simulink model "speedgoat_IO316_100k_21_CI_02826_v2"  (R2023a)
settings: Solver=FixedStepDiscrete  StartTime=0.0  StopTime=inf  RelTol=1e-3
PreLoadFcn:
  | if ~exist('Ts', 'var')
  | Ts = 0.001;
  | end
  | if ~exist('FPGA_Frequency', 'var')
  | FPGA_Frequency = 75000000;
  | end
  | if ~exist('Tpwm', 'var')
  | Tpwm = 0.005;
  | end
undefined symbols (not defined in the file or in its folder): IO316, IO3xx
libraries: simulink x3, speedgoatlib_fpga_pwm x2, speedgoatlib_fpga_dio x2, speedgoatlib_fpga_spi x2, hdlsllib x2, speedgoatlib_fpga_inta x1, speedgoatlib_interrupt x1, speedgoatlib_fpga_quadrature x1, speedgoatlib_fpga x1
settings Model: Creator=jeffrey.gruenig  LastModifiedBy=jeffrey.gruenig
settings SolverCC: ConcurrentTasks=on  PositivePriorityOrder=on
settings DataIOCC: SaveFormat=StructureWithTime
settings OptimizationCC: BlockReduction=off  OptimizeBlockIOStorage=off  BufferReuse=off
settings DebuggingCC: UnderspecifiedInitializationDetection=Classic  MergeDetectMultiDrivingBlocksExec=none  TasksWithSamePriorityMsg=none
settings HardwareCC: ProdBitPerLong=64  ProdLongLongMode=on  ProdHWDeviceType=Intel->x86-64 (Linux 64)
settings ModelReferenceCC: PropagateSignalLabelsOutOfModel=off
settings RTWCC: Description=Simulink Real-Time  SystemTargetFile=slrealtime.tlc  TemplateMakefile=slrealtime_default_tmf  Toolchain=Simulink Real-Time Toolchain  BuildConfiguration=Faster Runs  CodeExecutionProfiling=on  TargetLang=C++

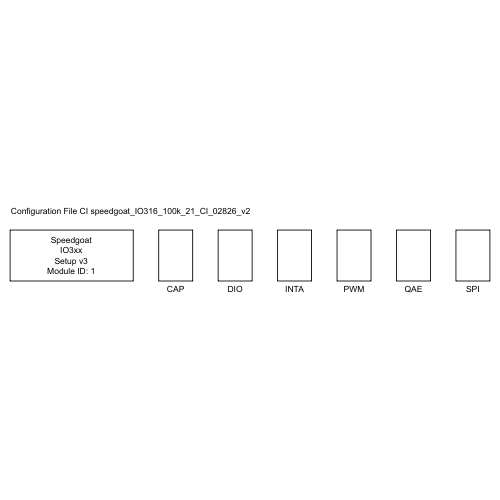
[thumbnail: Simulink's stored preview of the top-level diagram]
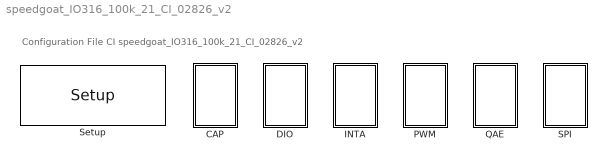
== system speedgoat_IO316_100k_21_CI_02826_v2 ==
  note: Configuration File CI speedgoat_IO316_100k_21_CI_02826_v2
  CAP : Subsystem
  DIO : Subsystem
  INTA : Subsystem
  PWM : Subsystem
  QAE : Subsystem
  SPI : Subsystem  Priority=1
  Setup : speedgoatlib_fpga/Setup/Setup  board=IO316-100k  id=1  device_id=1  frontIO=None  rearIO=IO3xx-21  bitstreamFile=speedgoat_IO316_100k_21_CI_02826_v2  rev=2.000000  timestamp_string=15/05/24 15:19:09  fpgaFreq=75 MHz  fpgaTick=13.33 ns  ProgSpiFlash=off  ProgBPIFlash=off  pciSlot=-1  useFpgaDmaController=off  PullRPort0=pull-up 3.3V  VioPort0=3.3V  PullRPort1=pull-up 3.3V  VioPort1=3.3V  PullRPort2=pull-up 3.3V  VioPort2=3.3V  PullRPort3=pull-up 3.3V  VioPort3=3.3V  PullRPort4=pull-up 3.3V  VioPort4=3.3V  PullRPort5=pull-up 3.3V  VioPort5=3.3V  PullRPort6=pull-up 3.3V  VioPort6=3.3V  diffLineTermination_rear1=on  diffLineTermination_rear2=on  diffLineTermination_rear3=on  diffLineTermination_rear4=on  diffLineTermination_rear5=on  diffLineTermination_rear6=on  diffLineTermination_rear7=on  diffLineTermination_rear8=on  PullRPort15=pull-up 3.3V  PullRPort31=pull-up 3.3V  PullRPort47=pull-up 3.3V  PullRPort63=pull-up 3.3V  diffLineTermination_1=on  diffLineTermination_2=on  diffLineTermination_3=on  diffLineTermination_4=on  diffLineTermination_5=on  diffLineTermination_6=on  diffLineTermination_7=on  diffLineTermination_8=on  diffLineTermination_9=on  diffLineTermination_10=on  diffLineTermination_11=on  diffLineTermination_12=on  diffLineTermination_13=on  diffLineTermination_14=on  diffLineTermination_15=on  diffLineTermination_16=on  diffLineTermination_17=on  diffLineTermination_18=on  diffLineTermination_19=on  diffLineTermination_20=on  diffLineTermination_21=on  diffLineTermination_22=on  diffLineTermination_23=on  diffLineTermination_24=on  diffLineTermination_25=on  diffLineTermination_26=on  diffLineTermination_27=on  diffLineTermination_28=on  diffLineTermination_29=on  diffLineTermination_30=on  diffLineTermination_31=on  diffLineTermination_32=on  Vo_36x_1=3.3V  Vi_Pull_36x_1=Floating  Vo_36x_2=3.3V  Vi_Pull_36x_2=Floating  Vo_36x_3=3.3V  Vi_Pull_36x_3=Floating  Vo_36x_4=3.3V  Vi_Pull_36x_4=Floating  Vo_36x_5=3.3V  Vi_Pull_36x_5=Floating  Vo_36x_6=3.3V  Vi_Pull_36x_6=Floating  Vo_36x_7=3.3V  Vi_Pull_36x_7=Floating  Vo_36x_8=3.3V  Vi_Pull_36x_8=Floating  Vo_36x_9_16=3.3V  Vi_Pull_36x_9_16=Floating  Vo_36x_17_24=3.3V  Vi_Pull_36x_17_24=Floating  Vo_36x_25_32=3.3V  Vi_Pull_36x_25_32=Floating  Vo_36x_33_40=3.3V  Vi_Pull_36x_33_40=Floating  Vo_36x_41_48=3.3V  Vi_Pull_36x_41_48=Floating  Vo_36x_49_56=3.3V  Vi_Pull_36x_49_56=Floating  Vo_36x_57_64=3.3V  Vi_Pull_36x_57_64=Floating
      settings: SourceProductName=Simulink Real-Time: Speedgoat I/O Blockset

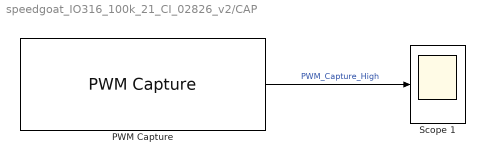
== system speedgoat_IO316_100k_21_CI_02826_v2/CAP ==
  PWM Capture : speedgoatlib_fpga_pwm/PWM Capture  id=1  chan=[1:2]  ts=Ts  enableDma=on  captureMode=High transitions triggered  bit_width_cap=24  captureTimeout_si=0  captureTimeout_eff=0  captureTimeout=0  debounce_si=10e-6  debounce_eff=10e-6  debounce=750  showHighDuration=off  showLowDuration=off  showPeriod=off  showDC16=on  showDC8=off  showTOn=off  showTOff=off  showValidData=off
      settings: SourceProductName=Simulink Real-Time: Speedgoat I/O Blockset
  "Scope 1 " : Scope
  wires:
  PWM Capture/1 -> "Scope 1 "/1  "PWM_Capture_High"

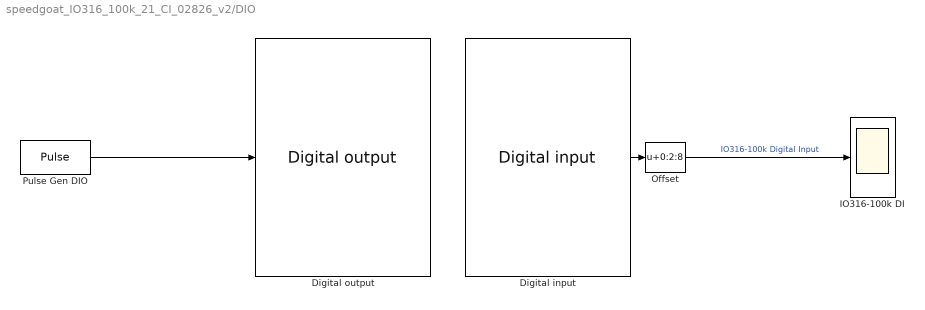
== system speedgoat_IO316_100k_21_CI_02826_v2/DIO ==
  Digital input : speedgoatlib_fpga_dio/Digital input  id=1  chan=[6,105:108]  ts=Ts  vectorizeOutput=on
      settings: SourceProductName=Simulink Real-Time: Speedgoat I/O Blockset
  Digital output : speedgoatlib_fpga_dio/Digital output  id=1  chan=[5,103:104]  init=[0]  reset=[0]  ts=Ts  vectorizeInput=on
      settings: SourceProductName=Simulink Real-Time: Speedgoat I/O Blockset
  IO316-100k DI : Scope
  Offset : Bias  Bias=0:2:8  SaturateOnIntegerOverflow=off
  Pulse Gen DIO : DiscretePulseGenerator  Period=20  PulseWidth=10  PhaseDelay=[0:5:10]  SampleTime=Ts  VectorParams1D=off
  wires:
  Offset/1 -> IO316-100k DI/1  "IO316-100k Digital Input"
  Digital input/1 -> Offset/1
  Pulse Gen DIO/1 -> Digital output/1

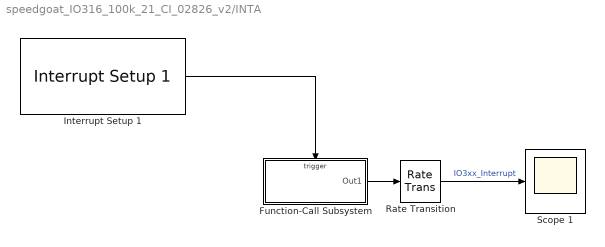
== system speedgoat_IO316_100k_21_CI_02826_v2/INTA ==
  Function-Call Subsystem : Subsystem  TreatAsAtomicUnit=on
  Interrupt Setup 1 : speedgoatlib_interrupt/Interrupt Setup 1  parModuleTrigger=off  parPollingMode=off  parPriorityConf=High  parPriority=241  confStartFcn=''  confStopFcn=''  confIsrFcn=''  confMapFcn=''  confHookFile=''  confIrqNr='-1'  confIsPolling=off  confModID='1'  confSelectedInt=Speedgoat IO316-100k interrupt  confSelectedId=1  confSelectedChannel=[]
  Rate Transition : RateTransition  Integrity=off
  "Scope 1 " : Scope
  wires:
  Rate Transition/1 -> "Scope 1 "/1  "IO3xx_Interrupt"
  Function-Call Subsystem/1(Out1) -> Rate Transition/1
  Interrupt Setup 1/1 -> Function-Call Subsystem/Trigger

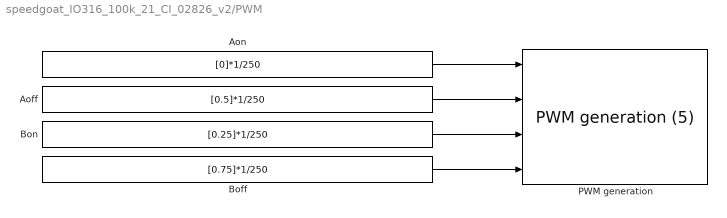
== system speedgoat_IO316_100k_21_CI_02826_v2/PWM ==
  Aoff : Constant  Value=[0.5]*1/250  OutDataTypeStr=Inherit: Inherit via back propagation  SampleTime=-1
  Aon : Constant  Value=[0]*1/250  VectorParams1D=off  OutDataTypeStr=Inherit: Inherit via back propagation  SampleTime=-1
  Boff : Constant  Value=[0.75]*1/250  OutDataTypeStr=Inherit: Inherit via back propagation  SampleTime=-1
  Bon : Constant  Value=[0.25]*1/250  OutDataTypeStr=Inherit: Inherit via back propagation  SampleTime=-1
  PWM generation : speedgoatlib_fpga_pwm/PWM generation (5)  id=1  chan=[1]  board=Please select...  ts=0.001  enableDma=off  pciSlot=-1  delay=0  symmetric=Asymmetric - On and Off are freely configurable  b_is_complement_of_a=Independent of PWM A output  deadband=[0.0]  period=[1/250]  frequency=250  ticks=74999  a_on=0  a_off=0.5e-3  pwm_a_dc=[0.0]  b_on=0.25e-3  b_off=0.75e-3  pwm_b_dc=[0]  c_on=[0.0]  c_off=[0.0]  protection=Disabled: A and B can be high at the same moment  enable_latch_half_period=off  pwm_update=At period starts  bit_width_pwm_gen=24  trigger_duration=[100e-6]  trigger_period_start=on  trigger_half_of_the_period=off  trigger_a_on=off  trigger_a_off=off  trigger_b_on=off  trigger_b_off=off  show_a_input=on  show_b_input=on  show_c_input=off  show_period_input=off  show_force_stop_input=off  idle_a=Low when PWM generation is halted  idle_b=Low when PWM generation is halted  idle_c=Low when PWM generation is halted  cancels_pwm_generation=on  invert_a=off  invert_b=off  invert_c=off
      settings: SourceProductName=Simulink Real-Time: Speedgoat I/O Blockset
  wires:
  Boff/1 -> PWM generation/4
  Bon/1 -> PWM generation/3
  Aoff/1 -> PWM generation/2
  Aon/1 -> PWM generation/1

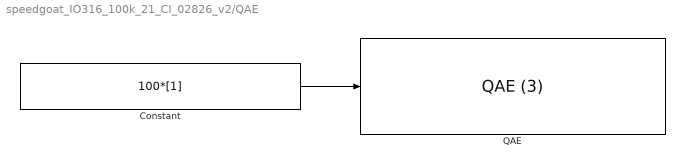
== system speedgoat_IO316_100k_21_CI_02826_v2/QAE ==
  Constant : Constant  Value=100*[1]
  QAE : speedgoatlib_fpga_quadrature/QAE (3)  id=1  chan=[1]  sampleTime=0.001  enableDma=on  numOfSlots=[16]  sigAswitchOn=[180]  sigBswitchOff=[90]  sigBswitchOn=[270]  initPos=0  sigAdismissEn=off  sigAdismissSingle=on  sigAdismissHigh=on  sigBdismissEn=off  sigBdismissSingle=on  sigBdismissHigh=on  showOutputPosition=off  showOutputSlotAngle=off
      settings: SourceProductName=Simulink Real-Time: Speedgoat I/O Blockset
  wires:
  Constant/1 -> QAE/1

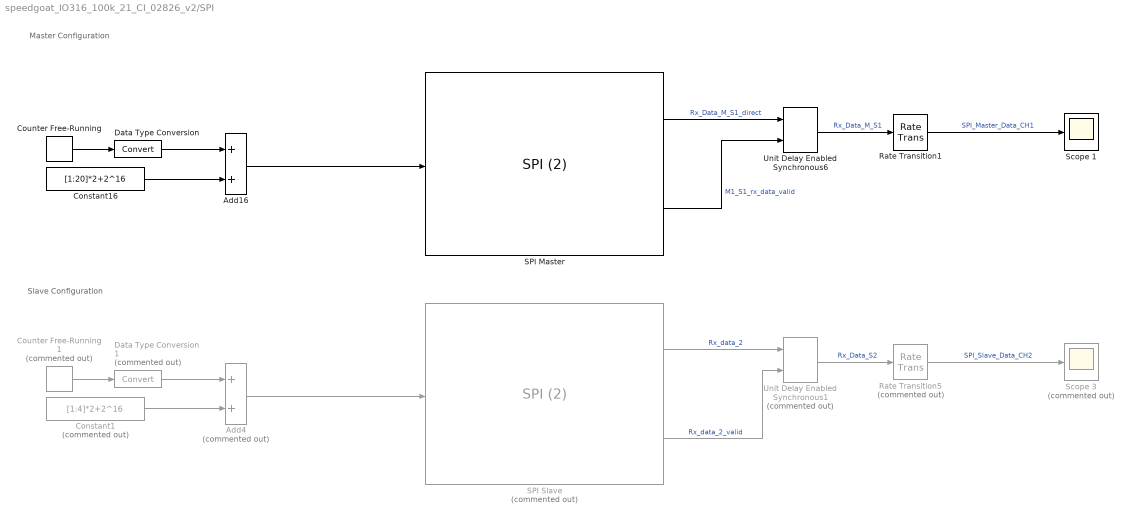
== system speedgoat_IO316_100k_21_CI_02826_v2/SPI ==
  note: Slave Configuration
  note: Master Configuration
  Add16 : Sum
  Add4 : Sum  Commented=on
  Constant1 : Constant  Commented=on  Value=[1:4]*2+2^16  OutDataTypeStr=Inherit: Inherit via back propagation
  Constant16 : Constant  Value=[1:20]*2+2^16  OutDataTypeStr=Inherit: Inherit via back propagation
  Counter Free-Running : simulink/Sources/Counter Free-Running  NumBits=32  tsamp=-1
  Counter Free-Running1 : simulink/Sources/Counter Free-Running  Commented=on  NumBits=32  tsamp=-1
  Data Type Conversion : DataTypeConversion  SaturateOnIntegerOverflow=off  RndMeth=Floor
  Data Type Conversion1 : DataTypeConversion  Commented=on  SaturateOnIntegerOverflow=off  RndMeth=Floor
  Rate Transition1 : RateTransition  Deterministic=off
  Rate Transition5 : RateTransition  Commented=on  Deterministic=off
  SPI Master : speedgoatlib_fpga_spi/SPI (2)  Priority=1  id=1  chan=[1]  samp_time=Ts*7  role=Master  sync_mode=off  multislave_mode=off  write_only=off  read_only=off  enableDma=off  multislave_chan=[1:8]  cpol=[0]  cpha=[1]  frequency=[350e3]  frequency_eff=350.5e3  delay_start=[2e-6]  delay_start_eff=2e-6  delay_interword=[2e-6]  delay_interword_eff=2e-6  delay_stop=[2e-6]  delay_stop_eff=2e-6  delay_compensation=[100e-9]  delay_compensation_eff=106.7e-9  words_per_frame=[20]  dynamic_words_per_frame=off  bits_per_word=[20]  bit_shift_lsb_first=[1]  no_cs=off  clock_timeout=[1e-6]  clock_timeout_eff=1E-06
      settings: SourceProductName=Simulink Real-Time: Speedgoat I/O Blockset
  SPI Slave : speedgoatlib_fpga_spi/SPI (2)  Commented=on  id=1  chan=[2]  samp_time=Ts*20  role=Slave  sync_mode=on  multislave_mode=off  write_only=off  read_only=off  enableDma=off  multislave_chan=[1]  cpol=[0]  cpha=[1]  frequency=[100e3]  frequency_eff=100000  delay_start=[1e-6]  delay_start_eff=1.06667E-07  delay_interword=[1e-6]  delay_interword_eff=1E-06  delay_stop=[1e-6]  delay_stop_eff=1E-06  delay_compensation=[1e-6]  delay_compensation_eff=1E-06  words_per_frame=[4]  dynamic_words_per_frame=off  bits_per_word=[20]  bit_shift_lsb_first=[1]  no_cs=off  clock_timeout=[10e-6]  clock_timeout_eff=1E-06
      settings: SourceProductName=Simulink Real-Time: Speedgoat I/O Blockset
  "Scope 1 " : Scope
  Scope 3 : Scope  Commented=on
  Unit Delay Enabled Synchronous1 : hdlsllib/Discrete/Unit Delay Enabled Synchronous  Commented=on  InitialCondition=0.0  SampleTime=-1
  Unit Delay Enabled Synchronous6 : hdlsllib/Discrete/Unit Delay Enabled Synchronous  InitialCondition=0.0  SampleTime=-1
  wires:
  Add16/1 -> SPI Master/1
  Rate Transition1/1 -> "Scope 1 "/1  "SPI_Master_Data_CH1"
  Add4/1 -> SPI Slave/1
  Constant1/1 -> Add4/2
  Constant16/1 -> Add16/2
  Data Type Conversion1/1 -> Add4/1
  SPI Slave/1 -> Unit Delay Enabled Synchronous1/1  "Rx_data_2"
  Unit Delay Enabled Synchronous1/1 -> Rate Transition5/1  "Rx_Data_S2"
  Counter Free-Running/1 -> Data Type Conversion/1
  SPI Slave/2 -> Unit Delay Enabled Synchronous1/2  "Rx_data_2_valid"
  SPI Master/2 -> Unit Delay Enabled Synchronous6/2  "M1_S1_rx_data_valid"
  SPI Master/1 -> Unit Delay Enabled Synchronous6/1  "Rx_Data_M_S1_direct"
  Data Type Conversion/1 -> Add16/1
  Rate Transition5/1 -> Scope 3/1  "SPI_Slave_Data_CH2"
  Unit Delay Enabled Synchronous6/1 -> Rate Transition1/1  "Rx_Data_M_S1"
  Counter Free-Running1/1 -> Data Type Conversion1/1

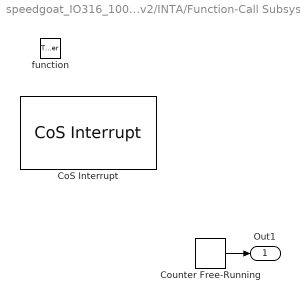
== system speedgoat_IO316_100k_21_CI_02826_v2/INTA/Function-Call Subsystem ==
  function : TriggerPort  TriggerType=function-call  VariantControl=Variant
  CoS Interrupt : speedgoatlib_fpga_inta/CoS Interrupt  id=1  ts=-1  debounce=0  delay=0  polarity=1
      settings: SourceProductName=Simulink Real-Time: Speedgoat I/O Blockset
  Counter Free-Running : simulink/Sources/Counter Free-Running  NumBits=32  tsamp=-1
  Out1 : Outport  InitialOutput=[0]  VectorParamsAs1DForOutWhenUnconnected=off
  wires:
  Counter Free-Running/1 -> Out1/1
